simulink model "Furnace"  (R2020a)
settings: Solver=ode15s  StartTime=0  StopTime=27000  FixedStep=0.1  MaxStep=20  MinStep=1e-13  RelTol=1e-08  AbsTol=1e-09
undefined symbols (not defined in the file): agnostic_lqe_params, cont_reg, disturbance_type, F_aI_pid, F_aII_pid, input_type, k, lqe_params, LQR_params, LQRAgnostic_params, MPC_type, MPCDiscrete_function_parameters, MPCDiscreteAgnostic_function_parameters, MPCDiscreteDiffIntegralAgnostic_function_parameters, original_LQR_params, output_type, reg, single_butter_ss
libraries: simulink x35, cstblocks x10, mpclib x3
(part 5 of 8)

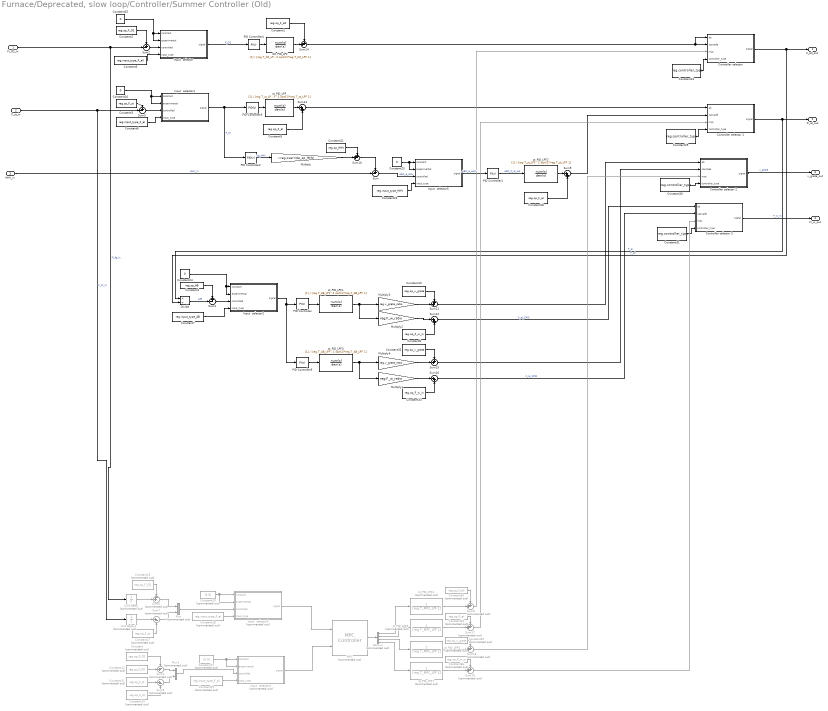
== system Furnace/Deprecated, slow loop/Controller/Summer Controller (Old)  ==
  Fi_O2_in : Inport
  F_st_in : Inport  Port=2
  HHV_in : Inport  Port=3
  Constant : Constant  Commented=on  Value=reg.op_F_O2
  Constant1 : Constant  Value=reg.op_F_aII
  Constant10 : Constant  Value=reg.op_v_grate
  Constant11 : Constant  Commented=on  Value=reg.sp_F_st
  Constant12 : Constant  Commented=on  Value=reg.sp_F_O2
  Constant{13,29..31} (4 alike) : Constant  Value=reg.controller_type
  Constant14 : Constant  Commented=on  Value=reg.op_F_st
  Constant15 : Constant  Commented=on  Value=reg.op_F_aI
  Constant16 : Constant  Commented=on  Value=reg.op_F_O2
  Constant17 : Constant  Commented=on  Value=reg.op_F_st
  Constant18 : Constant  Commented=on  Value=reg.input_type_F_aI
  Constant19 : Constant  Commented=on  Value=reg.input_type_F_aI
  Constant2 : Constant  Value=reg.sp_F_O2
  Constant20 : Constant  Commented=on  Value=[0 0]
  Constant21 : Constant  Value=reg.op_HHV
  Constant22 : Constant  Value=reg.input_type_HHV
  Constant{23..26} (4 alike) : Constant  Value=0
  Constant27 : Constant  Commented=on  Value=[0 0]
  Constant28 : Constant  Value=reg.op_F_aI
  Constant3 : Constant  Value=reg.sp_F_st
  Constant32 : Constant  Value=reg.op_v_grate
  Constant33 : Constant  Value=reg.op_F_w_in
  Constant34 : Constant  Commented=on  Value=reg.op_F_aII
  Constant35 : Constant  Commented=on  Value=reg.op_v_grate
  Constant36 : Constant  Commented=on  Value=reg.op_F_w_in
  Constant4 : Constant  Value=reg.sp_AB
  Constant5 : Constant  Value=reg.input_type_F_aII
  Constant6 : Constant  Value=reg.input_type_F_aI
  Constant7 : Constant  Value=reg.input_type_AB
  Constant8 : Constant  Value=reg.op_F_w_in
  Constant9 : Constant  Value=reg.op_F_aI
  "Controller selector " : MATLAB Function  TreatAsAtomicUnit=on
  Controller selector 1 : MATLAB Function  TreatAsAtomicUnit=on
  Controller selector 2 : MATLAB Function  TreatAsAtomicUnit=on
  Controller selector 3 : MATLAB Function  TreatAsAtomicUnit=on
  Demux : Demux  Commented=on
  Divide : Product  Inputs=*/  OutMin=[-100]  OutMax=[100]
  Input  selector : MATLAB Function  TreatAsAtomicUnit=on
  Input  selector1 : MATLAB Function  TreatAsAtomicUnit=on
  Input  selector2 : MATLAB Function  TreatAsAtomicUnit=on
  Input  selector3 : MATLAB Function  Commented=on  TreatAsAtomicUnit=on
  Input  selector4 : MATLAB Function  Commented=on  TreatAsAtomicUnit=on
  Input  selector5 : MATLAB Function  TreatAsAtomicUnit=on
  MPC : mpclib/MPC Controller  Commented=on  SCDEnableBlockLinearizationSpecification=on  mpcobj=lmpc  is_multiple=0  enable_value=0  return_u0=off  updateMPCinCallerWorkspace=on  md_inport=off  mv_inport=off  uref_inport=off  return_cost=off  return_mvseq=off  return_qpstatus=off  return_xseq=off  return_state=off  return_ovseq=off  state_inport=off  umin_inport=off  umax_inport=off  ymin_inport=off  ymax_inport=off  cc_inport=off  ywt_inport=off  uwt_inport=off  duwt_inport=off  rhoeps_inport=off  pm_inport=off  MaximumP=10  HorizonChoice=FixedHorizon  n_ts=20  n_p=50  n_mv=4  n_md=0  n_ud=0  n_mo=2  n_uo=0  BlockDataType=double  SampleTimeInherited=off  switch_inport=off
  Multiply : Gain  Gain=~reg.override_sp_HHV
  Multiply1 : Gain  Gain=reg.F_w_ratio
  Multiply2 : Gain  Gain=reg.F_w_ratio
  Multiply3 : Gain  Gain=reg.v_grate_ratio
  Multiply4 : Gain  Gain=reg.v_grate_ratio
  Mux : Mux  Commented=on  Inputs=2
  Mux1 : Mux  Commented=on  Inputs=2
  O2_PID_LPF : TransferFcn  Denominator=[reg.T_O2_LPF^2 sqrt(2)*reg.T_O2_LPF 1]
  PID Controller : simulink/Continuous/PID Controller  Controller=PI  Form=Parallel  TimeDomain=Discrete-time  UseExternalTs=off  SampleTime=1  IntegratorMethod=Forward Euler  FilterMethod=Forward Euler  ControllerParametersSource=internal  P=reg.Kp_AB  I=reg.Ki_AB  D=0  UseFilter=on  N=100  TunerSelectOption=Transfer Function Based (PID Tuner App)  InitialConditionSource=internal  InitialConditionForIntegrator=0  InitialConditionForFilter=0  DifferentiatorICPrevScaledInput=0  ExternalReset=none  TrackingMode=off  Kt=1  LimitOutput=off  UpperSaturationLimit=inf  LowerSaturationLimit=-inf  LinearizeAsGain=on  AntiWindupMode=none  Kb=1  POutMin=[]  POutMax=[]  IOutMin=[]  IOutMax=[]  DOutMin=[]  DOutMax=[]  NOutMin=[]  NOutMax=[]  SumOutMin=[]  SumOutMax=[]  SaturationOutMin=[]  SaturationOutMax=[]  PParamMin=[]  PParamMax=[]  IParamMin=[]  IParamMax=[]  DParamMin=[]  DParamMax=[]  NParamMin=[]  NParamMax=[]  KbParamMin=[]  KbParamMax=[]  KtParamMin=[]  KtParamMax=[]  KbOutMin=[]  KbOutMax=[]  KtOutMin=[]  KtOutMax=[]  IntegratorOutMin=[]  IntegratorOutMax=[]  FilterOutMin=[]  FilterOutMax=[]  SumI1OutMin=[]  SumI1OutMax=[]  SumI2OutMin=[]  SumI2OutMax=[]  SumI3OutMin=[]  SumI3OutMax=[]  SumI4OutMin=[]  SumI4OutMax=[]  SumDOutMin=[]  SumDOutMax=[]  DifferentiatorOutMin=[]  DifferentiatorOutMax=[]  FilterDiffOutCoefMin=[]  FilterDiffOutCoefMax=[]  ReciprocalOutMin=[]  ReciprocalOutMax=[]  SumDenOutMin=[]  SumDenOutMax=[]  SumNumOutMin=[]  SumNumOutMax=[]  DivideOutMin=[]  DivideOutMax=[]  UdiffTsProdOutMin=[]  UdiffTsProdOutMax=[]  NTsProdOutMin=[]  NTsProdOutMax=[]  UintegralTsProdOutMin=[]  UintegralTsProdOutMax=[]  UngainTsProdOutMin=[]  UngainTsProdOutMax=[]  IntegratorContinuousStateAttributes=''  IntegratorStateMustResolveToSignalObject=off  IntegratorRTWStateStorageClass=Auto  FilterContinuousStateAttributes=''  FilterStateMustResolveToSignalObject=off  FilterRTWStateStorageClass=Auto  ParallelPVariant=InternalParameters  IdealPVariant=Disabled  IVariant=InternalParameters  DVariant=Disabled  IntegratorVariant=Discrete  SatVariant=Disabled  AWVariant=Passthrough  PCopyVariant=Disabled  TRVariant=Disabled  FdbkBlocksVariant=Forward  IdealPFdbkVariant=Disabled  SatFdbkVariant=Disabled  DerivativeFilterVariant=Disabled  NVariant=Disabled  NCopyVariant=Disabled_SignalSpec  FilterICVariant=Disabled  IntegratorICVariant=InternalICs  ExternalResetVariant=Disabled  TRSumVariant=Passthrough  SumFdbkVariant=Disabled  SumVariant=Sum_PI  TsampFilterVariant=InternalTs  TsampNgainVariant=Passthrough  TsampIntegralVariant=Passthrough
  PID Controller1 : simulink/Continuous/PID Controller  Controller=PI  Form=Parallel  TimeDomain=Discrete-time  UseExternalTs=off  SampleTime=1  IntegratorMethod=Forward Euler  FilterMethod=Forward Euler  ControllerParametersSource=internal  P=reg.Kp_HHV  I=reg.Ki_HHV  D=0  UseFilter=on  N=100  TunerSelectOption=Transfer Function Based (PID Tuner App)  InitialConditionSource=internal  InitialConditionForIntegrator=0  InitialConditionForFilter=0  DifferentiatorICPrevScaledInput=0  ExternalReset=none  TrackingMode=off  Kt=1  LimitOutput=off  UpperSaturationLimit=inf  LowerSaturationLimit=-inf  LinearizeAsGain=on  AntiWindupMode=none  Kb=1  POutMin=[]  POutMax=[]  IOutMin=[]  IOutMax=[]  DOutMin=[]  DOutMax=[]  NOutMin=[]  NOutMax=[]  SumOutMin=[]  SumOutMax=[]  SaturationOutMin=[]  SaturationOutMax=[]  PParamMin=[]  PParamMax=[]  IParamMin=[]  IParamMax=[]  DParamMin=[]  DParamMax=[]  NParamMin=[]  NParamMax=[]  KbParamMin=[]  KbParamMax=[]  KtParamMin=[]  KtParamMax=[]  KbOutMin=[]  KbOutMax=[]  KtOutMin=[]  KtOutMax=[]  IntegratorOutMin=[]  IntegratorOutMax=[]  FilterOutMin=[]  FilterOutMax=[]  SumI1OutMin=[]  SumI1OutMax=[]  SumI2OutMin=[]  SumI2OutMax=[]  SumI3OutMin=[]  SumI3OutMax=[]  SumI4OutMin=[]  SumI4OutMax=[]  SumDOutMin=[]  SumDOutMax=[]  DifferentiatorOutMin=[]  DifferentiatorOutMax=[]  FilterDiffOutCoefMin=[]  FilterDiffOutCoefMax=[]  ReciprocalOutMin=[]  ReciprocalOutMax=[]  SumDenOutMin=[]  SumDenOutMax=[]  SumNumOutMin=[]  SumNumOutMax=[]  DivideOutMin=[]  DivideOutMax=[]  UdiffTsProdOutMin=[]  UdiffTsProdOutMax=[]  NTsProdOutMin=[]  NTsProdOutMax=[]  UintegralTsProdOutMin=[]  UintegralTsProdOutMax=[]  UngainTsProdOutMin=[]  UngainTsProdOutMax=[]  IntegratorContinuousStateAttributes=''  IntegratorStateMustResolveToSignalObject=off  IntegratorRTWStateStorageClass=Auto  FilterContinuousStateAttributes=''  FilterStateMustResolveToSignalObject=off  FilterRTWStateStorageClass=Auto  ParallelPVariant=InternalParameters  IdealPVariant=Disabled  IVariant=InternalParameters  DVariant=Disabled  IntegratorVariant=Discrete  SatVariant=Disabled  AWVariant=Passthrough  PCopyVariant=Disabled  TRVariant=Disabled  FdbkBlocksVariant=Forward  IdealPFdbkVariant=Disabled  SatFdbkVariant=Disabled  DerivativeFilterVariant=Disabled  NVariant=Disabled  NCopyVariant=Disabled_SignalSpec  FilterICVariant=Disabled  IntegratorICVariant=InternalICs  ExternalResetVariant=Disabled  TRSumVariant=Passthrough  SumFdbkVariant=Disabled  SumVariant=Sum_PI  TsampFilterVariant=InternalTs  TsampNgainVariant=Passthrough  TsampIntegralVariant=Passthrough
  PID Controller2 : simulink/Continuous/PID Controller  Controller=PID  Form=Parallel  TimeDomain=Discrete-time  UseExternalTs=off  SampleTime=1  IntegratorMethod=Forward Euler  FilterMethod=Forward Euler  ControllerParametersSource=internal  P=reg.Kp_st_HHV  I=reg.Ki_st_HHV  D=reg.Kd_st_HHV  UseFilter=on  N=100  TunerSelectOption=Transfer Function Based (PID Tuner App)  InitialConditionSource=internal  InitialConditionForIntegrator=0.001  InitialConditionForFilter=0  DifferentiatorICPrevScaledInput=0  ExternalReset=none  TrackingMode=off  Kt=1  LimitOutput=off  UpperSaturationLimit=inf  LowerSaturationLimit=1  LinearizeAsGain=on  AntiWindupMode=none  Kb=1  POutMin=[]  POutMax=[]  IOutMin=[]  IOutMax=[]  DOutMin=[]  DOutMax=[]  NOutMin=[]  NOutMax=[]  SumOutMin=[]  SumOutMax=[]  SaturationOutMin=[]  SaturationOutMax=[]  PParamMin=[]  PParamMax=[]  IParamMin=[]  IParamMax=[]  DParamMin=[]  DParamMax=[]  NParamMin=[]  NParamMax=[]  KbParamMin=[]  KbParamMax=[]  KtParamMin=[]  KtParamMax=[]  KbOutMin=[]  KbOutMax=[]  KtOutMin=[]  KtOutMax=[]  IntegratorOutMin=[]  IntegratorOutMax=[]  FilterOutMin=[]  FilterOutMax=[]  SumI1OutMin=[]  SumI1OutMax=[]  SumI2OutMin=[]  SumI2OutMax=[]  SumI3OutMin=[]  SumI3OutMax=[]  SumI4OutMin=[]  SumI4OutMax=[]  SumDOutMin=[]  SumDOutMax=[]  DifferentiatorOutMin=[]  DifferentiatorOutMax=[]  FilterDiffOutCoefMin=[]  FilterDiffOutCoefMax=[]  ReciprocalOutMin=[]  ReciprocalOutMax=[]  SumDenOutMin=[]  SumDenOutMax=[]  SumNumOutMin=[]  SumNumOutMax=[]  DivideOutMin=[]  DivideOutMax=[]  UdiffTsProdOutMin=[]  UdiffTsProdOutMax=[]  NTsProdOutMin=[]  NTsProdOutMax=[]  UintegralTsProdOutMin=[]  UintegralTsProdOutMax=[]  UngainTsProdOutMin=[]  UngainTsProdOutMax=[]  IntegratorContinuousStateAttributes='F_st'  IntegratorStateMustResolveToSignalObject=off  IntegratorRTWStateStorageClass=Auto  FilterContinuousStateAttributes=''  FilterStateMustResolveToSignalObject=off  FilterRTWStateStorageClass=Auto  ParallelPVariant=InternalParameters  IdealPVariant=Disabled  IVariant=InternalParameters  DVariant=InternalParameters  IntegratorVariant=Discrete  SatVariant=Disabled  AWVariant=Passthrough  PCopyVariant=Disabled  TRVariant=Disabled  FdbkBlocksVariant=Forward  IdealPFdbkVariant=Disabled  SatFdbkVariant=Disabled  DerivativeFilterVariant=ForwardEulerFilter  NVariant=InternalParameters  NCopyVariant=Disabled  FilterICVariant=InternalICsFilter  IntegratorICVariant=InternalICs  ExternalResetVariant=Disabled  TRSumVariant=Passthrough  SumFdbkVariant=Disabled  SumVariant=Sum_PID  TsampFilterVariant=InternalTs  TsampNgainVariant=Passthrough  TsampIntegralVariant=Passthrough
  PID Controller3 : simulink/Continuous/PID Controller  Controller=PID  Form=Parallel  TimeDomain=Discrete-time  UseExternalTs=off  SampleTime=1  IntegratorMethod=Forward Euler  FilterMethod=Forward Euler  ControllerParametersSource=internal  P=reg.Kp_st  I=reg.Ki_st  D=reg.Kd_st  UseFilter=on  N=100  TunerSelectOption=Transfer Function Based (PID Tuner App)  InitialConditionSource=internal  InitialConditionForIntegrator=0  InitialConditionForFilter=0  DifferentiatorICPrevScaledInput=0  ExternalReset=none  TrackingMode=off  Kt=1  LimitOutput=off  UpperSaturationLimit=inf  LowerSaturationLimit=1  LinearizeAsGain=on  AntiWindupMode=none  Kb=1  POutMin=[]  POutMax=[]  IOutMin=[]  IOutMax=[]  DOutMin=[]  DOutMax=[]  NOutMin=[]  NOutMax=[]  SumOutMin=[]  SumOutMax=[]  SaturationOutMin=[]  SaturationOutMax=[]  PParamMin=[]  PParamMax=[]  IParamMin=[]  IParamMax=[]  DParamMin=[]  DParamMax=[]  NParamMin=[]  NParamMax=[]  KbParamMin=[]  KbParamMax=[]  KtParamMin=[]  KtParamMax=[]  KbOutMin=[]  KbOutMax=[]  KtOutMin=[]  KtOutMax=[]  IntegratorOutMin=[]  IntegratorOutMax=[]  FilterOutMin=[]  FilterOutMax=[]  SumI1OutMin=[]  SumI1OutMax=[]  SumI2OutMin=[]  SumI2OutMax=[]  SumI3OutMin=[]  SumI3OutMax=[]  SumI4OutMin=[]  SumI4OutMax=[]  SumDOutMin=[]  SumDOutMax=[]  DifferentiatorOutMin=[]  DifferentiatorOutMax=[]  FilterDiffOutCoefMin=[]  FilterDiffOutCoefMax=[]  ReciprocalOutMin=[]  ReciprocalOutMax=[]  SumDenOutMin=[]  SumDenOutMax=[]  SumNumOutMin=[]  SumNumOutMax=[]  DivideOutMin=[]  DivideOutMax=[]  UdiffTsProdOutMin=[]  UdiffTsProdOutMax=[]  NTsProdOutMin=[]  NTsProdOutMax=[]  UintegralTsProdOutMin=[]  UintegralTsProdOutMax=[]  UngainTsProdOutMin=[]  UngainTsProdOutMax=[]  IntegratorContinuousStateAttributes='F_st'  IntegratorStateMustResolveToSignalObject=off  IntegratorRTWStateStorageClass=Auto  FilterContinuousStateAttributes=''  FilterStateMustResolveToSignalObject=off  FilterRTWStateStorageClass=Auto  ParallelPVariant=InternalParameters  IdealPVariant=Disabled  IVariant=InternalParameters  DVariant=InternalParameters  IntegratorVariant=Discrete  SatVariant=Disabled  AWVariant=Passthrough  PCopyVariant=Disabled  TRVariant=Disabled  FdbkBlocksVariant=Forward  IdealPFdbkVariant=Disabled  SatFdbkVariant=Disabled  DerivativeFilterVariant=ForwardEulerFilter  NVariant=InternalParameters  NCopyVariant=Disabled  FilterICVariant=InternalICsFilter  IntegratorICVariant=InternalICs  ExternalResetVariant=Disabled  TRSumVariant=Passthrough  SumFdbkVariant=Disabled  SumVariant=Sum_PID  TsampFilterVariant=InternalTs  TsampNgainVariant=Passthrough  TsampIntegralVariant=Passthrough
  PID Controller4 : simulink/Continuous/PID Controller  Controller=PI  Form=Parallel  TimeDomain=Discrete-time  UseExternalTs=off  SampleTime=1  IntegratorMethod=Forward Euler  FilterMethod=Forward Euler  ControllerParametersSource=internal  P=reg.Kp_O2  I=reg.Ki_O2  D=0  UseFilter=on  N=100  TunerSelectOption=Transfer Function Based (PID Tuner App)  InitialConditionSource=internal  InitialConditionForIntegrator=0.001  InitialConditionForFilter=0  DifferentiatorICPrevScaledInput=0  ExternalReset=none  TrackingMode=off  Kt=1  LimitOutput=off  UpperSaturationLimit=inf  LowerSaturationLimit=1  LinearizeAsGain=on  AntiWindupMode=none  Kb=1  POutMin=[]  POutMax=[]  IOutMin=[]  IOutMax=[]  DOutMin=[]  DOutMax=[]  NOutMin=[]  NOutMax=[]  SumOutMin=[]  SumOutMax=[]  SaturationOutMin=[]  SaturationOutMax=[]  PParamMin=[]  PParamMax=[]  IParamMin=[]  IParamMax=[]  DParamMin=[]  DParamMax=[]  NParamMin=[]  NParamMax=[]  KbParamMin=[]  KbParamMax=[]  KtParamMin=[]  KtParamMax=[]  KbOutMin=[]  KbOutMax=[]  KtOutMin=[]  KtOutMax=[]  IntegratorOutMin=[]  IntegratorOutMax=[]  FilterOutMin=[]  FilterOutMax=[]  SumI1OutMin=[]  SumI1OutMax=[]  SumI2OutMin=[]  SumI2OutMax=[]  SumI3OutMin=[]  SumI3OutMax=[]  SumI4OutMin=[]  SumI4OutMax=[]  SumDOutMin=[]  SumDOutMax=[]  DifferentiatorOutMin=[]  DifferentiatorOutMax=[]  FilterDiffOutCoefMin=[]  FilterDiffOutCoefMax=[]  ReciprocalOutMin=[]  ReciprocalOutMax=[]  SumDenOutMin=[]  SumDenOutMax=[]  SumNumOutMin=[]  SumNumOutMax=[]  DivideOutMin=[]  DivideOutMax=[]  UdiffTsProdOutMin=[]  UdiffTsProdOutMax=[]  NTsProdOutMin=[]  NTsProdOutMax=[]  UintegralTsProdOutMin=[]  UintegralTsProdOutMax=[]  UngainTsProdOutMin=[]  UngainTsProdOutMax=[]  IntegratorContinuousStateAttributes='F_st'  IntegratorStateMustResolveToSignalObject=off  IntegratorRTWStateStorageClass=Auto  FilterContinuousStateAttributes=''  FilterStateMustResolveToSignalObject=off  FilterRTWStateStorageClass=Auto  ParallelPVariant=InternalParameters  IdealPVariant=Disabled  IVariant=InternalParameters  DVariant=Disabled  IntegratorVariant=Discrete  SatVariant=Disabled  AWVariant=Passthrough  PCopyVariant=Disabled  TRVariant=Disabled  FdbkBlocksVariant=Forward  IdealPFdbkVariant=Disabled  SatFdbkVariant=Disabled  DerivativeFilterVariant=Disabled  NVariant=Disabled  NCopyVariant=Disabled_SignalSpec  FilterICVariant=Disabled  IntegratorICVariant=InternalICs  ExternalResetVariant=Disabled  TRSumVariant=Passthrough  SumFdbkVariant=Disabled  SumVariant=Sum_PI  TsampFilterVariant=InternalTs  TsampNgainVariant=Passthrough  TsampIntegralVariant=Passthrough
  PID Controller5 : simulink/Continuous/PID Controller  Controller=PI  Form=Parallel  TimeDomain=Discrete-time  UseExternalTs=off  SampleTime=1  IntegratorMethod=Forward Euler  FilterMethod=Forward Euler  ControllerParametersSource=internal  P=reg.Kp_AB_HHV  I=reg.Ki_AB_HHV  D=0  UseFilter=on  N=100  TunerSelectOption=Transfer Function Based (PID Tuner App)  InitialConditionSource=internal  InitialConditionForIntegrator=0  InitialConditionForFilter=0  DifferentiatorICPrevScaledInput=0  ExternalReset=none  TrackingMode=off  Kt=1  LimitOutput=off  UpperSaturationLimit=inf  LowerSaturationLimit=-inf  LinearizeAsGain=on  AntiWindupMode=none  Kb=1  POutMin=[]  POutMax=[]  IOutMin=[]  IOutMax=[]  DOutMin=[]  DOutMax=[]  NOutMin=[]  NOutMax=[]  SumOutMin=[]  SumOutMax=[]  SaturationOutMin=[]  SaturationOutMax=[]  PParamMin=[]  PParamMax=[]  IParamMin=[]  IParamMax=[]  DParamMin=[]  DParamMax=[]  NParamMin=[]  NParamMax=[]  KbParamMin=[]  KbParamMax=[]  KtParamMin=[]  KtParamMax=[]  KbOutMin=[]  KbOutMax=[]  KtOutMin=[]  KtOutMax=[]  IntegratorOutMin=[]  IntegratorOutMax=[]  FilterOutMin=[]  FilterOutMax=[]  SumI1OutMin=[]  SumI1OutMax=[]  SumI2OutMin=[]  SumI2OutMax=[]  SumI3OutMin=[]  SumI3OutMax=[]  SumI4OutMin=[]  SumI4OutMax=[]  SumDOutMin=[]  SumDOutMax=[]  DifferentiatorOutMin=[]  DifferentiatorOutMax=[]  FilterDiffOutCoefMin=[]  FilterDiffOutCoefMax=[]  ReciprocalOutMin=[]  ReciprocalOutMax=[]  SumDenOutMin=[]  SumDenOutMax=[]  SumNumOutMin=[]  SumNumOutMax=[]  DivideOutMin=[]  DivideOutMax=[]  UdiffTsProdOutMin=[]  UdiffTsProdOutMax=[]  NTsProdOutMin=[]  NTsProdOutMax=[]  UintegralTsProdOutMin=[]  UintegralTsProdOutMax=[]  UngainTsProdOutMin=[]  UngainTsProdOutMax=[]  IntegratorContinuousStateAttributes=''  IntegratorStateMustResolveToSignalObject=off  IntegratorRTWStateStorageClass=Auto  FilterContinuousStateAttributes=''  FilterStateMustResolveToSignalObject=off  FilterRTWStateStorageClass=Auto  ParallelPVariant=InternalParameters  IdealPVariant=Disabled  IVariant=InternalParameters  DVariant=Disabled  IntegratorVariant=Discrete  SatVariant=Disabled  AWVariant=Passthrough  PCopyVariant=Disabled  TRVariant=Disabled  FdbkBlocksVariant=Forward  IdealPFdbkVariant=Disabled  SatFdbkVariant=Disabled  DerivativeFilterVariant=Disabled  NVariant=Disabled  NCopyVariant=Disabled_SignalSpec  FilterICVariant=Disabled  IntegratorICVariant=InternalICs  ExternalResetVariant=Disabled  TRSumVariant=Passthrough  SumFdbkVariant=Disabled  SumVariant=Sum_PI  TsampFilterVariant=InternalTs  TsampNgainVariant=Passthrough  TsampIntegralVariant=Passthrough
  Sum{,2..4} (4 alike) : Sum  Inputs=+-|
  Sum1 : Sum  Commented=on  Inputs=-+|
  Sum{10..11,14..15} (4 alike) : Sum  Inputs=++|
  Sum{9,12..13,16} (4 alike) : Sum  Inputs=|++
  Sum{8,17..19} (4 alike) : Sum  Commented=on  Inputs=++|
  Sum5 : Sum  Commented=on  Inputs=|+-
  Sum6 : Sum  Commented=on  Inputs=-+|
  Sum7 : Sum  Commented=on  Inputs=|+-
  Unit Delay : UnitDelay  Commented=on  HasFrameUpgradeWarning=on
  Unit Delay1 : UnitDelay  Commented=on  HasFrameUpgradeWarning=on
  st_PID_LPF : TransferFcn  Denominator=[reg.T_st_LPF^2 sqrt(2)*reg.T_st_LPF 1]
  st_PID_LPF1 : TransferFcn  Denominator=[reg.T_AB_LPF^2 sqrt(2)*reg.T_AB_LPF 1]
  st_PID_LPF2 : TransferFcn  Denominator=[reg.T_st_LPF^2 sqrt(2)*reg.T_st_LPF 1]
  st_PID_LPF3 : TransferFcn  Denominator=[reg.T_AB_LPF^2 sqrt(2)*reg.T_AB_LPF 1]
  st_PID_LPF{4..7} (4 alike) : TransferFcn  Commented=on  Denominator=[reg.T_MPC_LPF 1]
  F_aII_out : Outport  VectorParamsAs1DForOutWhenUnconnected=off
  Fi_aI_out : Outport  Port=2  VectorParamsAs1DForOutWhenUnconnected=off
  v_grate_out : Outport  Port=3  VectorParamsAs1DForOutWhenUnconnected=off
  Fi_w_out : Outport  Port=4  VectorParamsAs1DForOutWhenUnconnected=off
  wires:
  Input  selector/1(signal) -> PID Controller4/1  "F_O2"
  Constant7/1 -> Input  selector2/4(input_type)
  Constant5/1 -> Input  selector/4(input_type)
  Constant4/1 -> Sum4/1
  Fi_O2_in/1 -> Unit Delay/1, Sum2/2  "Fi_fg_in"
  Constant2/1 -> Sum2/1
  F_st_in/1 -> Sum3/2, Unit Delay1/1  "F_st_in"
  Constant3/1 -> Sum3/1
  PID Controller4/1 -> O2_PID_LPF/1
  Sum14/1 -> "Controller selector "/1(ab), "Controller selector "/2(cascade)
  PID Controller3/1 -> st_PID_LPF/1
  Sum13/1 -> Controller selector 1/1(ab)
  Constant8/1 -> Sum12/2
  PID Controller/1 -> st_PID_LPF1/1
  Sum11/1 -> Controller selector 2/1(ab)
  Multiply2/1 -> Sum12/1
  Constant10/1 -> Sum11/1
  st_PID_LPF/1 -> Sum13/1
  st_PID_LPF1/1 -> Multiply2/1, Multiply3/1
  Demux/1 -> st_PID_LPF4/1
  Demux/2 -> st_PID_LPF5/1
  Demux/3 -> st_PID_LPF6/1
  Demux/4 -> st_PID_LPF7/1
  "Controller selector "/1(signal) -> Divide/2, F_aII_out/1  "F_aII"
  Controller selector 1/1(signal) -> Divide/1, Fi_aI_out/1  "F_aI"
  Controller selector 2/1(signal) -> v_grate_out/1  "v_grate"
  Controller selector 3/1(signal) -> Fi_w_out/1  "F_w_in"
  Constant12/1 -> Sum1/2
  Constant/1 -> Sum1/1
  Constant11/1 -> Sum5/1
  Constant14/1 -> Sum5/2
  Sum5/1 -> Mux1/2
  MPC/1 -> Demux/1
  Sum7/1 -> Mux/2
  Constant16/1 -> Sum6/1
  Constant17/1 -> Sum7/2
  Input  selector3/1(signal) -> MPC/1
  Mux/1 -> Input  selector3/3(controlled)
  Constant18/1 -> Input  selector3/4(input_type)
  Constant19/1 -> Input  selector4/4(input_type)
  Mux1/1 -> Input  selector4/3(controlled)
  Input  selector4/1(signal) -> MPC/2
  Constant20/1 -> Input  selector3/2(experimental), Input  selector3/1(constant)
  HHV_in/1 -> Sum/2  "HHV_in"
  Input  selector5/1(signal) -> PID Controller1/1  "ABC_e_HHV"
  Constant22/1 -> Input  selector5/4(input_type)
  Sum/1 -> Input  selector5/3(controlled)  "ABC_e_HHV"
  Constant23/1 -> Input  selector5/2(experimental), Input  selector5/1(constant)
  Divide/1 -> Sum4/2  "A/B"
  Sum4/1 -> Input  selector2/3(controlled)
  Input  selector2/1(signal) -> PID Controller5/1, PID Controller/1
  Constant24/1 -> Input  selector2/2(experimental), Input  selector2/1(constant)
  Sum2/1 -> Input  selector/3(controlled)
  Constant25/1 -> Input  selector/2(experimental), Input  selector/1(constant)
  Sum3/1 -> Input  selector1/3(controlled)
  Constant6/1 -> Input  selector1/4(input_type)
  Constant26/1 -> Input  selector1/2(experimental), Input  selector1/1(constant)
  Input  selector1/1(signal) -> PID Controller3/1, PID Controller2/1  "F_st"
  Constant27/1 -> Input  selector4/2(experimental), Input  selector4/1(constant)
  Sum12/1 -> Controller selector 3/1(ab)  "F_aI_CPID"
  PID Controller1/1 -> st_PID_LPF2/1  "ABC_F_aI_out"
  Sum9/1 -> Controller selector 1/2(cascade)
  PID Controller2/1 -> Multiply/1  "sp_HHV"
  Multiply/1 -> Sum10/2
  Constant21/1 -> Sum10/1
  Sum10/1 -> Sum/1
  st_PID_LPF2/1 -> Sum9/1
  Sum1/1 -> Mux1/1
  Sum6/1 -> Mux/1
  Constant28/1 -> Sum9/2
  Constant9/1 -> Sum13/2
  O2_PID_LPF/1 -> Sum14/2
  Constant1/1 -> Sum14/1
  Constant13/1 -> "Controller selector "/4(controller_type)
  Constant29/1 -> Controller selector 1/4(controller_type)
  Constant30/1 -> Controller selector 2/4(controller_type)
  Constant31/1 -> Controller selector 3/4(controller_type)
  st_PID_LPF3/1 -> Multiply1/1, Multiply4/1
  PID Controller5/1 -> st_PID_LPF3/1
  Constant33/1 -> Sum16/2
  Constant32/1 -> Sum15/1
  Multiply1/1 -> Sum16/1
  Sum15/1 -> Controller selector 2/2(cascade)
  Sum16/1 -> Controller selector 3/2(cascade)  "F_aI_CPID"
  Unit Delay/1 -> Sum6/2
  Unit Delay1/1 -> Sum7/1
  st_PID_LPF4/1 -> Sum8/2
  st_PID_LPF5/1 -> Sum17/2
  st_PID_LPF6/1 -> Sum18/2
  st_PID_LPF7/1 -> Sum19/2
  Constant34/1 -> Sum8/1
  Constant15/1 -> Sum17/1
  Constant35/1 -> Sum18/1
  Constant36/1 -> Sum19/1
  Sum17/1 -> Controller selector 1/3(mpc)
  Sum8/1 -> "Controller selector "/3(mpc)
  Sum18/1 -> Controller selector 2/3(mpc)
  Sum19/1 -> Controller selector 3/3(mpc)
  Multiply3/1 -> Sum11/2
  Multiply4/1 -> Sum15/2

== system Furnace/Deprecated, slow loop/Furnace/Ashes ==
  In1 : Inport
  In2 : Inport  Port=2
  In Bus Element : Inport  Port=3  PortName=InBus  Element=M_w_grate
  In Bus Element1 : Inport  Port=3  PortName=InBus  Element=M_char
  In Bus Element2 : Inport  Port=3  PortName=InBus  Element=F_w_ash
  In Bus Element3 : Inport  Port=3  PortName=InBus  Element=F_char_ash
  Flow of char ash : Display
  Flow of waste ash : Display
  Mass of char in grate : Display
  Scope1 : Scope
  Sum of Elements : Sum  Inputs=+  CollapseMode=Specified dimension
  Temperatures in grate : Display
  Waste in grate (mass) : Display
  wires:
  In Bus Element2/1 -> Flow of waste ash/1
  In Bus Element/1 -> Waste in grate (mass)/1
  In Bus Element1/1 -> Mass of char in grate/1
  In Bus Element3/1 -> Flow of char ash/1
  In1/1 -> Sum of Elements/1
  In2/1 -> Temperatures in grate/1
  Sum of Elements/1 -> Scope1/1

== system Furnace/Deprecated, slow loop/Furnace/Auxiliary "burners" ==
  In1 : Inport
  Constant : Constant  Value=0
  Constant1 : Constant  Value=850+k.T_amb
  Minus : Sum  Inputs=+-
  "Q " : Constant  Value=3.5e6
  Switch : Switch  Criteria=u2 > Threshold
  Out1 : Outport  VectorParamsAs1DForOutWhenUnconnected=off
  wires:
  Switch/1 -> Out1/1
  Constant/1 -> Switch/3
  "Q "/1 -> Switch/1
  Minus/1 -> Switch/2
  Constant1/1 -> Minus/1
  In1/1 -> Minus/2

== system Furnace/Deprecated, slow loop/Furnace/Boiler ==
  T_fromHE : Inport
  T_fg : Inport  Port=2
  F_fg : Inport  Port=3
  F_flyash : Inport  Port=4
  F_ECO : Inport  Port=5
  Constant : Constant  Value=0
  Constant1 : Constant  Value=k.p_drum
  Constant2 : Constant  Value=k.p_drum
  Drum : Subsystem
      mask Display: image('Drum.jpg');
  Economizer : Subsystem
  Evaporator : Subsystem
  Gain : Gain  Gain=1e-5
  Goto : Goto  Commented=on  GotoTag=T_drum  TagVisibility=global
  MATLAB Function : MATLAB Function  TreatAsAtomicUnit=on
  PID Controller : simulink/Continuous/PID Controller  Controller=PID  Form=Parallel  TimeDomain=Continuous-time  UseExternalTs=off  SampleTime=-1  IntegratorMethod=Forward Euler  FilterMethod=Forward Euler  ControllerParametersSource=internal  P=10  I=0  D=0  UseFilter=on  N=100  TunerSelectOption=Transfer Function Based (PID Tuner App)  InitialConditionSource=internal  InitialConditionForIntegrator=0  InitialConditionForFilter=0  DifferentiatorICPrevScaledInput=0  ExternalReset=none  TrackingMode=off  Kt=1  LimitOutput=on  UpperSaturationLimit=50  LowerSaturationLimit=0  LinearizeAsGain=on  AntiWindupMode=none  Kb=1  POutMin=[]  POutMax=[]  IOutMin=[]  IOutMax=[]  DOutMin=[]  DOutMax=[]  NOutMin=[]  NOutMax=[]  SumOutMin=[]  SumOutMax=[]  SaturationOutMin=[]  SaturationOutMax=[]  PParamMin=[]  PParamMax=[]  IParamMin=[]  IParamMax=[]  DParamMin=[]  DParamMax=[]  NParamMin=[]  NParamMax=[]  KbParamMin=[]  KbParamMax=[]  KtParamMin=[]  KtParamMax=[]  KbOutMin=[]  KbOutMax=[]  KtOutMin=[]  KtOutMax=[]  IntegratorOutMin=[]  IntegratorOutMax=[]  FilterOutMin=[]  FilterOutMax=[]  SumI1OutMin=[]  SumI1OutMax=[]  SumI2OutMin=[]  SumI2OutMax=[]  SumI3OutMin=[]  SumI3OutMax=[]  SumI4OutMin=[]  SumI4OutMax=[]  SumDOutMin=[]  SumDOutMax=[]  DifferentiatorOutMin=[]  DifferentiatorOutMax=[]  FilterDiffOutCoefMin=[]  FilterDiffOutCoefMax=[]  ReciprocalOutMin=[]  ReciprocalOutMax=[]  SumDenOutMin=[]  SumDenOutMax=[]  SumNumOutMin=[]  SumNumOutMax=[]  DivideOutMin=[]  DivideOutMax=[]  UdiffTsProdOutMin=[]  UdiffTsProdOutMax=[]  NTsProdOutMin=[]  NTsProdOutMax=[]  UintegralTsProdOutMin=[]  UintegralTsProdOutMax=[]  UngainTsProdOutMin=[]  UngainTsProdOutMax=[]  IntegratorContinuousStateAttributes=''  IntegratorStateMustResolveToSignalObject=off  IntegratorRTWStateStorageClass=Auto  FilterContinuousStateAttributes=''  FilterStateMustResolveToSignalObject=off  FilterRTWStateStorageClass=Auto  ParallelPVariant=InternalParameters  IdealPVariant=Disabled  IVariant=InternalParameters  DVariant=InternalParameters  IntegratorVariant=Continuous  SatVariant=Enabled  AWVariant=Passthrough  PCopyVariant=Disabled  TRVariant=Disabled  FdbkBlocksVariant=Forward  IdealPFdbkVariant=Disabled  SatFdbkVariant=Disabled  DerivativeFilterVariant=ContFilter  NVariant=InternalParameters  NCopyVariant=Disabled  FilterICVariant=InternalICsFilter  IntegratorICVariant=InternalICs  ExternalResetVariant=Disabled  TRSumVariant=Passthrough  SumFdbkVariant=Disabled  SumVariant=Sum_PID  TsampFilterVariant=InternalTs  TsampNgainVariant=Passthrough  TsampIntegralVariant=Passthrough
  PID null saturator : Switch
  Scope : Scope
  Scope1 : Scope
  Scope2 : Scope
  Sum1 : Sum  Inputs=+-|
  Super heater : Subsystem
  x_vap : Scope
  T_SH : Outport  VectorParamsAs1DForOutWhenUnconnected=off
  F_SH : Outport  Port=2  PortDimensions=1  VectorParamsAs1DForOutWhenUnconnected=off
  p_drum : Outport  Port=3  VectorParamsAs1DForOutWhenUnconnected=off
  T_fg_out : Outport  Port=4  VectorParamsAs1DForOutWhenUnconnected=off
  Fi_fg_out : Outport  Port=5  VectorParamsAs1DForOutWhenUnconnected=off
  F_flyash_out : Outport  Port=6  VectorParamsAs1DForOutWhenUnconnected=off
  wires:
  Evaporator/3(Fi_fg_out) -> Super heater/4(Fi_fg)
  Super heater/4(Fi_fg_out) -> Economizer/3(Fi_fg)
  Super heater/3(T_fg_out) -> Economizer/2(T_fg)
  Evaporator/2(T_fg_out) -> Super heater/3(T_fg)
  Economizer/3(Fi_fg_out) -> Fi_fg_out/1
  F_fg/1 -> Evaporator/3(Fi_fg)
  T_fg/1 -> Evaporator/2(T_fg)
  Super heater/2(T_steam) -> T_SH/1
  Economizer/2(T_fg_out) -> T_fg_out/1
  Drum/3(p_drum) -> MATLAB Function/1(p_drum), Sum1/1, p_drum/1
  T_fromHE/1 -> Economizer/1(T_fromHE)
  Super heater/5(F_SH) -> F_SH/1
  Drum/2(x_vap) -> x_vap/1
  PID Controller/1 -> Drum/3(F_vap), Scope/1, Super heater/1(F_steam)
  Constant1/1 -> Sum1/2
  Constant/1 -> PID null saturator/3
  Sum1/1 -> Gain/1
  [Q_cleaning] -> Drum/5(Q_cleaning)
  F_flyash/1 -> F_flyash_out/1
  Super heater/1(Q_SH) -> Scope1/1
  Economizer/1(Q_ECO) -> Scope2/1
  Economizer/4(F_ECO) -> Drum/1(F_ECO)
  Evaporator/1(Q_EVA) -> Drum/2(Q_EVA)
  Economizer/5(T_ECO2) -> Drum/4(T_ECO)
  F_ECO/1 -> Economizer/4(F_w)
  PID null saturator/1 -> PID Controller/1
  Gain/1 -> PID null saturator/1
  Drum/1(T_drum) -> Goto/1, Super heater/2(T_drum), Evaporator/1(T_drum)
  MATLAB Function/1(switch_on) -> PID null saturator/2
  Constant2/1 -> MATLAB Function/2(k_p_drum)

== system Furnace/Deprecated, slow loop/Furnace/Calorific Value ==
  T_fg : Inport
  Fi_fg : Inport  Port=2
  From : From  Commented=on  GotoTag=F_aII
  From1 : From  Commented=on  GotoTag=T_aI  TagVisibility=global
  From2 : From  Commented=on  GotoTag=F_aI  TagVisibility=global
  From3 : From  Commented=on  GotoTag=T_aII
  MATLAB Function : MATLAB Function  TreatAsAtomicUnit=on
  T_amb : Constant  Value=k.T_amb
  cp_fg : Constant  Value=k.cp_fg
  HHV : Outport  VectorParamsAs1DForOutWhenUnconnected=off
  wires:
  cp_fg/1 -> MATLAB Function/3(cp_fg)
  Fi_fg/1 -> MATLAB Function/1(Fi_fg)
  T_amb/1 -> MATLAB Function/4(T_amb)
  MATLAB Function/1(HHV) -> HHV/1
  T_fg/1 -> MATLAB Function/2(T_fg)
  From2/1 -> MATLAB Function/5(F_aI)
  From1/1 -> MATLAB Function/6(T_aI)
  From/1 -> MATLAB Function/7(F_aII)
  From3/1 -> MATLAB Function/8(T_aII)

== system Furnace/Deprecated, slow loop/Furnace/Cold water from district heating ==
  Constant : Constant  Value=reg.const_F_from_DH
  Constant2 : Constant  Value=reg.const_T_from_DH
  From Workspace1 : FromWorkspace  VariableName=F_from_DH
  From Workspace2 : FromWorkspace  VariableName=T_from_DH
  Selector : Selector  InputPortWidth=2  IndexOptions=Index vector (dialog)  Indices=reg.input_type_F_from_DH  OutputSizes=1
  Selector1 : Selector  InputPortWidth=2  IndexOptions=Index vector (dialog)  Indices=reg.input_type_T_from_DH  OutputSizes=1
  Vector Concatenate : Concatenate
  Vector Concatenate1 : Concatenate
  Out1 : Outport  VectorParamsAs1DForOutWhenUnconnected=off
  Out2 : Outport  Port=2  VectorParamsAs1DForOutWhenUnconnected=off
  wires:
  From Workspace1/1 -> Vector Concatenate/2
  Constant/1 -> Vector Concatenate/1
  Constant2/1 -> Vector Concatenate1/1
  From Workspace2/1 -> Vector Concatenate1/2
  Vector Concatenate/1 -> Selector/1
  Selector/1 -> Out1/1  "F_from_DH"
  Vector Concatenate1/1 -> Selector1/1
  Selector1/1 -> Out2/1  "T_from_DH"

== system Furnace/Deprecated, slow loop/Furnace/Condenser ==
  F_district : Inport
  F_turb : Inport  Port=2
  T_return : Inport  Port=3
  Constant : Constant  Value=k.cp_water
  Constant1 : Constant  Value=k.epsilon_HE
  Constant2 : Constant  Value=k.eff_HE
  District heating heat exchanger : MATLAB Function  TreatAsAtomicUnit=on
  Scope : Scope
  Transport Delay1 : TransportDelay  DelayTime=2
  Transport Delay2 : TransportDelay  DelayTime=2  InitialOutput=k.T_amb  BufferSize=2048
  Transport Delay3 : TransportDelay  DelayTime=2  InitialOutput=k.T_amb
  Transport Delay4 : TransportDelay  DelayTime=2  InitialOutput=k.T_amb
  p_HP : Constant  Value=k.p_HP
  T_district : Outport  VectorParamsAs1DForOutWhenUnconnected=off
  T_w_out : Outport  Port=2  VectorParamsAs1DForOutWhenUnconnected=off
  F_cond : Outport  Port=3  VectorParamsAs1DForOutWhenUnconnected=off
  wires:
  F_district/1 -> District heating heat exchanger/1(F_DH)
  p_HP/1 -> District heating heat exchanger/2(p_HP)
  T_return/1 -> District heating heat exchanger/4(T_return)
  Constant/1 -> District heating heat exchanger/5(cp_water)
  Constant1/1 -> District heating heat exchanger/6(epsilon_HE)
  District heating heat exchanger/1(Q_HE) -> Transport Delay1/1
  District heating heat exchanger/3(T_district) -> Transport Delay3/1
  District heating heat exchanger/2(Tw_ECO) -> Transport Delay2/1
  F_turb/1 -> Transport Delay4/1, District heating heat exchanger/3(F_turb)
  Transport Delay1/1 -> Scope/1
  Transport Delay2/1 -> T_w_out/1
  Transport Delay3/1 -> T_district/1
  Constant2/1 -> District heating heat exchanger/7(eff_HE)
  Transport Delay4/1 -> F_cond/1

== system Furnace/Deprecated, slow loop/Furnace/Flue-gas fan ==
  T_fg : Inport
  Fi_fg : Inport  Port=2
  Fan : MATLAB Function  TreatAsAtomicUnit=on
  Sum of Elements : Sum  Inputs=+
  Out1 : Outport  VectorParamsAs1DForOutWhenUnconnected=off
  Out2 : Outport  Port=2  VectorParamsAs1DForOutWhenUnconnected=off
  tag scope: W_fan=global
  wires:
  T_fg/1 -> Fan/1(T_fg)
  Sum of Elements/1 -> Fan/2(F_fg)
  Fi_fg/1 -> Out2/1, Sum of Elements/1
  Fan/1(T_out) -> Out1/1
  Fan/2(W_el) -> [W_fan]

== system Furnace/Deprecated, slow loop/Furnace/Flue-gas stack ==
  T_fg : Inport
  Fi_fg : Inport  Port=2
  F_fg : Scope
  T_fg_fromECO : Scope
  wires:
  T_fg/1 -> T_fg_fromECO/1
  Fi_fg/1 -> F_fg/1

== system Furnace/Deprecated, slow loop/Furnace/Free board ==
  Fi_in : Inport
  T_in : Inport  Port=2
  Q_rad : Inport  Port=3
  F_flyash_cell : Inport  Port=4
  F_aII_in : Inport  Port=5
  T_aII_in : Inport  Port=6
  DIFF_Free Board : MATLAB Function  TreatAsAtomicUnit=on
  M_fg_part : Integrator  InitialCondition=[k.M_fg_IC.*k.w_a(1:k.nc_gas-1)]
  M_steel : Constant  Value=k.M_steel_FB
  Mw_gas : Constant  Value=k.Mw_gas
  Scope : Scope
  Sum of Elements : Sum  Inputs=+
  T_amb : Constant  Value=k.T_amb
  T_fg : Integrator  InitialCondition=k.T_0
  To Workspace : ToWorkspace  Commented=on  VariableName=Y_H2O  SaveFormat=Structure With Time  SampleTime=-1
  V_FB : Constant  Value=k.V_FreeBoard
  cp_fg : Constant  Value=k.cp_fg
  cp_steel : Constant  Value=k.cp_steel
  p_amb : Constant  Value=k.p_amb
  T_fg_out : Outport  VectorParamsAs1DForOutWhenUnconnected=off
  Fi_fg_to_boiler : Outport  Port=2  VectorParamsAs1DForOutWhenUnconnected=off
  F_flyash_tot : Outport  Port=3  VectorParamsAs1DForOutWhenUnconnected=off
  wires:
  T_in/1 -> DIFF_Free Board/4(T_in)  "T_in"
  p_amb/1 -> DIFF_Free Board/8(p_amb)
  DIFF_Free Board/1(dMfg_dt_int) -> M_fg_part/1
  DIFF_Free Board/2(dTfg_dt) -> T_fg/1
  M_fg_part/1 -> DIFF_Free Board/1(M_fg_int)
  DIFF_Free Board/4(M_fg) -> Scope/1
  Q_rad/1 -> DIFF_Free Board/7(Q_rad)  "Q_rad"
  Fi_in/1 -> DIFF_Free Board/3(Fi_in)
  DIFF_Free Board/5(Y_H2O) -> To Workspace/1
  T_fg/1 -> DIFF_Free Board/2(T_fg), T_fg_out/1
  DIFF_Free Board/3(Fi_fg_out) -> Fi_fg_to_boiler/1
  V_FB/1 -> DIFF_Free Board/9(V_FreeBoard)
  Mw_gas/1 -> DIFF_Free Board/10(Mw_gas)
  T_amb/1 -> DIFF_Free Board/11(T_amb)
  cp_fg/1 -> DIFF_Free Board/12(cp_fg)
  cp_steel/1 -> DIFF_Free Board/13(cp_steel)
  M_steel/1 -> DIFF_Free Board/14(M_steel_FB)
  F_flyash_cell/1 -> Sum of Elements/1
  Sum of Elements/1 -> F_flyash_tot/1
  F_aII_in/1 -> DIFF_Free Board/5(F_aII)
  T_aII_in/1 -> DIFF_Free Board/6(T_aII)

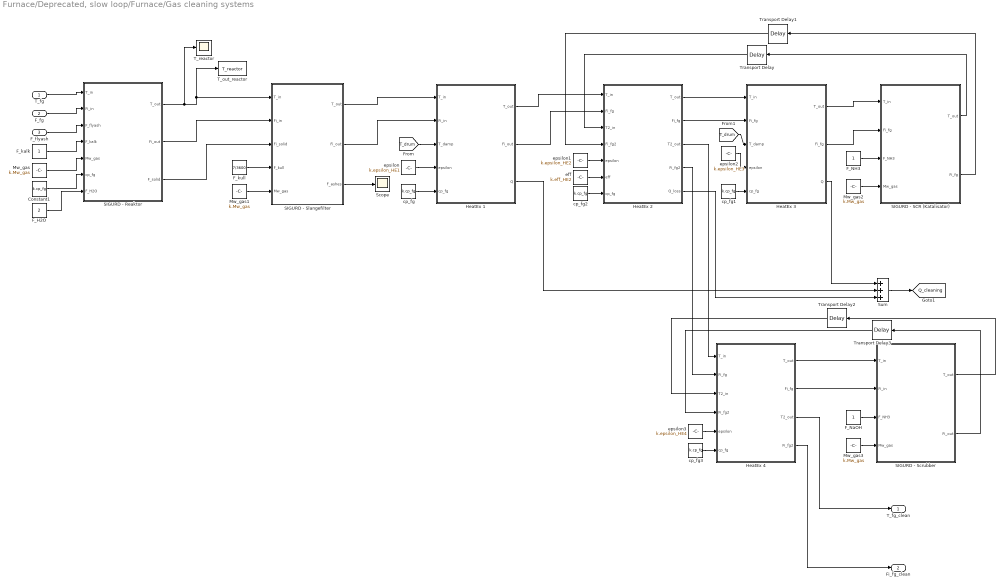
== system Furnace/Deprecated, slow loop/Furnace/Gas cleaning systems ==
  T_fg : Inport
  F_fg : Inport  Port=2
  F_flyash : Inport  Port=3
  Constant1 : Constant  Value=k.cp_fg
  F_H2O : Constant  Value=2
  F_NH3 : Constant
  F_NaOH : Constant
  F_kalk : Constant
  F_kull : Constant  Value=7/3600
  HeatEx 1 : MATLAB Function  TreatAsAtomicUnit=on
  HeatEx 2 : MATLAB Function  TreatAsAtomicUnit=on
  HeatEx 3 : MATLAB Function  TreatAsAtomicUnit=on
  HeatEx 4 : MATLAB Function  TreatAsAtomicUnit=on
  Mw_gas{,1..3} (4 alike) : Constant  Value=k.Mw_gas
  SIGURD - Reaktor : MATLAB Function  TreatAsAtomicUnit=on
  SIGURD - SCR (Katalisator) : MATLAB Function  TreatAsAtomicUnit=on
  SIGURD - Scrubber : MATLAB Function  TreatAsAtomicUnit=on
  SIGURD - Slangefilter : MATLAB Function  TreatAsAtomicUnit=on
  Scope : Scope
  Sum : Sum  Inputs=+++
  T_out_reactor : ToWorkspace  VariableName=T_reactor  SaveFormat=Timeseries  SampleTime=-1
  T_reactor : Scope
  Transport Delay : TransportDelay  DelayTime=2  InitialOutput=k.T_amb
  Transport Delay1 : TransportDelay  DelayTime=2  InitialOutput=ones(k.nc_gas,1)
  Transport Delay2 : TransportDelay  DelayTime=2  InitialOutput=k.T_amb
  Transport Delay3 : TransportDelay  DelayTime=2  InitialOutput=ones(k.nc_gas,1)
  cp_fg{,1..3} (4 alike) : Constant  Value=k.cp_fg
  eff : Constant  Value=k.eff_HE2
  epsilon : Constant  Value=k.epsilon_HE1
  epsilon1 : Constant  Value=k.epsilon_HE2
  epsilon2 : Constant  Value=k.epsilon_HE3
  epsilon3 : Constant  Value=k.epsilon_HE4
  T_fg_clean : Outport  VectorParamsAs1DForOutWhenUnconnected=off
  Fi_fg_clean : Outport  Port=2  VectorParamsAs1DForOutWhenUnconnected=off
  tag scope: Q_cleaning=global
  wires:
  T_fg/1 -> SIGURD - Reaktor/1(T_in)
  F_fg/1 -> SIGURD - Reaktor/2(Fi_in)
  SIGURD - Reaktor/1(T_out) -> T_reactor/1, T_out_reactor/1, SIGURD - Slangefilter/1(T_in)
  SIGURD - Reaktor/2(Fi_out) -> SIGURD - Slangefilter/2(Fi_in)
  F_kalk/1 -> SIGURD - Reaktor/4(F_kalk)
  Mw_gas/1 -> SIGURD - Reaktor/5(Mw_gas)
  F_kull/1 -> SIGURD - Slangefilter/4(F_kull)
  Mw_gas1/1 -> SIGURD - Slangefilter/5(Mw_gas)
  SIGURD - Slangefilter/1(T_out) -> HeatEx 1/1(T_in)
  SIGURD - Slangefilter/2(Fi_out) -> HeatEx 1/2(Fi_in)
  [T_drum] -> HeatEx 1/3(T_damp)
  epsilon/1 -> HeatEx 1/4(epsilon)
  HeatEx 1/1(T_out) -> HeatEx 2/1(T_in)
  HeatEx 1/2(Fi_out) -> HeatEx 2/2("Fi_fg ")
  HeatEx 2/1(T_out) -> HeatEx 3/1(T_in)
  HeatEx 2/2(Fi_fg) -> HeatEx 3/2("Fi_fg ")
  [T_drum] -> HeatEx 3/3(T_damp)
  epsilon1/1 -> HeatEx 2/5(epsilon)
  epsilon2/1 -> HeatEx 3/4(epsilon)
  HeatEx 1/3(Q) -> Sum/2
  HeatEx 3/3(Q) -> Sum/1
  HeatEx 3/1(T_out) -> SIGURD - SCR (Katalisator)/1(T_in)
  HeatEx 3/2(Fi_fg) -> SIGURD - SCR (Katalisator)/2("Fi_fg ")
  F_NH3/1 -> SIGURD - SCR (Katalisator)/3(F_NH3)
  Mw_gas2/1 -> SIGURD - SCR (Katalisator)/4(Mw_gas)
  SIGURD - SCR (Katalisator)/1(T_out) -> Transport Delay/1
  SIGURD - SCR (Katalisator)/2(Fi_fg) -> Transport Delay1/1
  HeatEx 2/3(T2_out) -> HeatEx 4/1(T_in)
  HeatEx 2/4(Fi_fg2) -> HeatEx 4/2("Fi_fg ")
  epsilon3/1 -> HeatEx 4/5(epsilon)
  HeatEx 4/1(T_out) -> SIGURD - Scrubber/1(T_in)
  HeatEx 4/2(Fi_fg) -> SIGURD - Scrubber/2(Fi_in)
  SIGURD - Scrubber/1(T_out) -> Transport Delay2/1
  SIGURD - Scrubber/2(Fi_out) -> Transport Delay3/1
  F_NaOH/1 -> SIGURD - Scrubber/3(F_NH3)
  Mw_gas3/1 -> SIGURD - Scrubber/4(Mw_gas)
  HeatEx 4/3(T2_out) -> T_fg_clean/1
  HeatEx 4/4(Fi_fg2) -> Fi_fg_clean/1
  SIGURD - Slangefilter/3(F_ashes) -> Scope/1
  cp_fg/1 -> HeatEx 1/5(cp_fg)
  cp_fg1/1 -> HeatEx 3/5(cp_fg)
  cp_fg2/1 -> HeatEx 2/7(cp_fg)
  Constant1/1 -> SIGURD - Reaktor/6(cp_fg)
  SIGURD - Reaktor/3(F_solid) -> SIGURD - Slangefilter/3(Fi_solid)
  F_flyash/1 -> SIGURD - Reaktor/3(F_flyash)
  Transport Delay/1 -> HeatEx 2/3(T2_in)
  Transport Delay1/1 -> HeatEx 2/4("Fi_fg2 ")
  Transport Delay2/1 -> HeatEx 4/3(T2_in)
  Transport Delay3/1 -> HeatEx 4/4("Fi_fg2 ")
  cp_fg3/1 -> HeatEx 4/6(cp_fg)
  eff/1 -> HeatEx 2/6(eff)
  Sum/1 -> [Q_cleaning]
  HeatEx 2/5(Q_loss) -> Sum/3
  F_H2O/1 -> SIGURD - Reaktor/7(F_H2O)

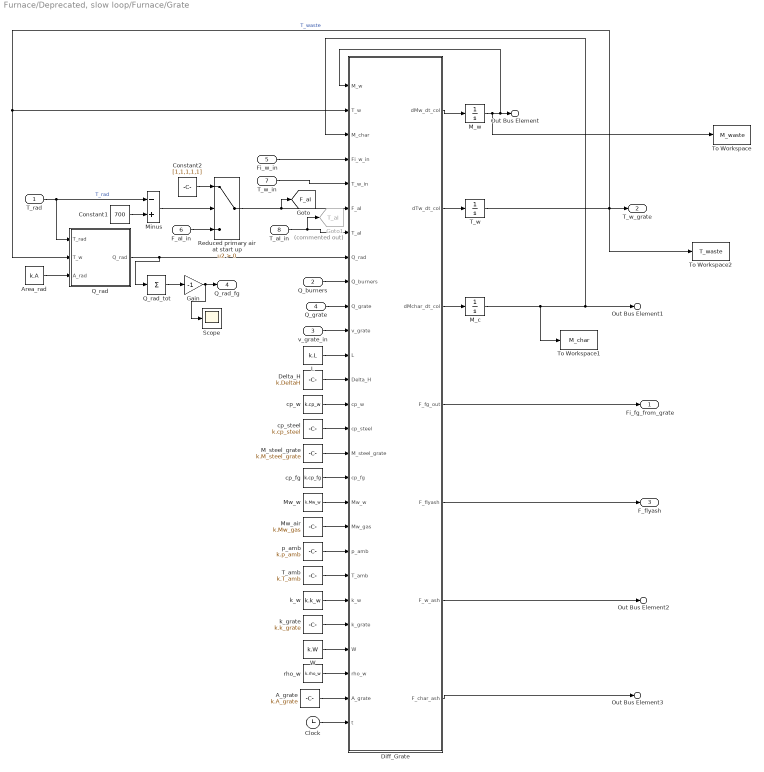
== system Furnace/Deprecated, slow loop/Furnace/Grate ==
  T_rad : Inport
  Q_burners : Inport  Port=2
  v_grate_in : Inport  Port=3
  Q_grate : Inport  Port=4
  Fi_w_in : Inport  Port=5
  F_aI_in : Inport  Port=6
  T_w_in : Inport  Port=7
  T_aI_in : Inport  Port=8
  A_grate : Constant  Value=k.A_grate
  Area_rad : Constant  Value=k.A
  Clock : Clock
  Constant1 : Constant  Value=700
  Constant2 : Constant  Value=[1,1,1,1,1]
  Delta_H : Constant  Value=k.DeltaH
  Diff_Grate : MATLAB Function  TreatAsAtomicUnit=on
  Gain : Gain  Gain=-1
  Goto1 : Goto  Commented=on  GotoTag=T_aI  TagVisibility=global
  L : Constant  Value=k.L
  M_c : Integrator  InitialCondition=zeros(k.n_cell,1)
  M_steel_grate : Constant  Value=k.M_steel_grate
  M_w : Integrator  InitialCondition=zeros(k.n_cell.*(k.nc_w+2),1)
  Minus : Sum  Inputs=-+
  Mw_air : Constant  Value=k.Mw_gas
  Mw_w : Constant  Value=k.Mw_w
  Q_rad : Subsystem
  Q_rad_tot : Sum  Inputs=+
  Reduced primary air at start up : Switch  Criteria=u2 > Threshold
  Scope : Scope
  T_amb : Constant  Value=k.T_amb
  T_w : Integrator  InitialCondition=k.T_amb.*ones(k.n_cell,1)
  To Workspace : ToWorkspace  VariableName=M_waste  SaveFormat=Structure With Time  SampleTime=-1
  To Workspace1 : ToWorkspace  VariableName=M_char  SaveFormat=Structure With Time  SampleTime=-1
  To Workspace2 : ToWorkspace  VariableName=T_waste  SaveFormat=Structure With Time  SampleTime=-1
  W : Constant  Value=k.W
  cp_fg : Constant  Value=k.cp_fg
  cp_steel : Constant  Value=k.cp_steel
  cp_w : Constant  Value=k.cp_w
  k_grate : Constant  Value=k.k_grate
  k_w : Constant  Value=k.k_w
  p_amb : Constant  Value=k.p_amb
  rho_w : Constant  Value=k.rho_w
  Fi_fg_from_grate : Outport  VectorParamsAs1DForOutWhenUnconnected=off
  T_w_grate : Outport  Port=2  VectorParamsAs1DForOutWhenUnconnected=off
  F_flyash : Outport  Port=3  VectorParamsAs1DForOutWhenUnconnected=off
  Q_rad_fg : Outport  Port=4  VectorParamsAs1DForOutWhenUnconnected=off
  Out Bus Element : Outport  Port=5  VectorParamsAs1DForOutWhenUnconnected=off  PortName=OutBus  Element=M_w_grate
  Out Bus Element1 : Outport  Port=5  VectorParamsAs1DForOutWhenUnconnected=off  PortName=OutBus  Element=M_char
  Out Bus Element2 : Outport  Port=5  VectorParamsAs1DForOutWhenUnconnected=off  PortName=OutBus  Element=F_w_ash
  Out Bus Element3 : Outport  Port=5  VectorParamsAs1DForOutWhenUnconnected=off  PortName=OutBus  Element=F_char_ash
  tag scope: F_aI=global
  wires:
  Diff_Grate/2(dTw_dt_col) -> T_w/1
  Area_rad/1 -> Q_rad/3(A_rad)
  M_w/1 -> To Workspace/1, Out Bus Element/1, Diff_Grate/1(M_w)
  T_aI_in/1 -> Goto1/1, Diff_Grate/7(T_aI)
  Q_rad/1(Q_rad) -> Q_rad_tot/1, Diff_Grate/8(Q_rad)
  Diff_Grate/1(dMw_dt_col) -> M_w/1
  T_w/1 -> Diff_Grate/2(T_w), Q_rad/2(T_w), T_w_grate/1, To Workspace2/1  "T_waste"
  Diff_Grate/6(F_w_ash) -> Out Bus Element2/1
  Diff_Grate/4(F_fg_out) -> Fi_fg_from_grate/1
  Diff_Grate/3(dMchar_dt_col) -> M_c/1
  M_c/1 -> To Workspace1/1, Out Bus Element1/1, Diff_Grate/3(M_char)
  Diff_Grate/7(F_char_ash) -> Out Bus Element3/1
  Q_rad_tot/1 -> Gain/1
  Gain/1 -> Scope/1, Q_rad_fg/1
  Q_burners/1 -> Diff_Grate/9(Q_burners)
  Clock/1 -> Diff_Grate/27(t)
  Q_grate/1 -> Diff_Grate/10(Q_grate)
  T_rad/1 -> Minus/1, Q_rad/1(T_rad)  "T_rad"
  Constant1/1 -> Minus/2
  Minus/1 -> Reduced primary air at start up/2
  F_aI_in/1 -> Reduced primary air at start up/3
  Reduced primary air at start up/1 -> [F_aI], Diff_Grate/6(F_aI)
  Constant2/1 -> Reduced primary air at start up/1
  L/1 -> Diff_Grate/12(L)
  Delta_H/1 -> Diff_Grate/13(Delta_H)
  cp_w/1 -> Diff_Grate/14(cp_w)
  cp_steel/1 -> Diff_Grate/15(cp_steel)
  M_steel_grate/1 -> Diff_Grate/16(M_steel_grate)
  cp_fg/1 -> Diff_Grate/17(cp_fg)
  Mw_w/1 -> Diff_Grate/18(Mw_w)
  Mw_air/1 -> Diff_Grate/19(Mw_gas)
  p_amb/1 -> Diff_Grate/20(p_amb)
  T_amb/1 -> Diff_Grate/21(T_amb)
  k_w/1 -> Diff_Grate/22(k_w)
  k_grate/1 -> Diff_Grate/23(k_grate)
  W/1 -> Diff_Grate/24(W)
  rho_w/1 -> Diff_Grate/25(rho_w)
  A_grate/1 -> Diff_Grate/26(A_grate)
  Diff_Grate/5(F_flyash) -> F_flyash/1
  v_grate_in/1 -> Diff_Grate/11(v_grate)
  Fi_w_in/1 -> Diff_Grate/4(Fi_w_in)
  T_w_in/1 -> Diff_Grate/5(T_w_in)

== system Furnace/Deprecated, slow loop/Furnace/Hot water to district heating ==
  In1 : Inport
  T_district : Scope
  wires:
  In1/1 -> T_district/1

== system Furnace/Deprecated, slow loop/Furnace/Turbine ==
  T_SH : Inport
  F_SH : Inport  Port=2
  p_drum : Inport  Port=3
  Scope : Scope
  Sum : Sum
  Transport Delay1 : TransportDelay  DelayTime=3
  Transport Delay2 : TransportDelay  DelayTime=3
  Turbine : MATLAB Function  TreatAsAtomicUnit=on
  W_net : Scope
  eta_TURB : Constant  Value=k.eta_TURB
  p_HP : Constant  Value=k.p_HP
  p_LP : Constant  Value=k.p_LP
  F_turb : Outport  VectorParamsAs1DForOutWhenUnconnected=off
  wires:
  T_SH/1 -> Turbine/1(T_SH)
  Turbine/1(W_el) -> Transport Delay1/1
  p_drum/1 -> Turbine/3(p_drum)
  F_SH/1 -> Transport Delay2/1, Turbine/2(F_SH)
  p_LP/1 -> Turbine/5(p_LP)
  Transport Delay1/1 -> Sum/1
  Transport Delay2/1 -> F_turb/1
  p_HP/1 -> Turbine/4(p_HP)
  Turbine/2(Q_turb) -> Scope/1
  eta_TURB/1 -> Turbine/6(eta_TURB)
  [W_fan] -> Sum/2
  Sum/1 -> W_net/1

== system Furnace/Plant2/Boiler/Drum ==
  F_ECO : Inport
  Q_EVA : Inport  Port=2
  F_vap : Inport  Port=3
  T_ECO : Inport  Port=4
  Q_cleaning : Inport  Port=5
  Constant : Constant  Value=k.p_amb
  Constant1 : Constant  Value=k.T_amb
  Constant10 : Constant  Value=k.cp_fg
  Constant11 : Constant  Value=k.Mw_air
  Constant2 : Constant  Value=k.Mw_water
  Constant3 : Constant  Value=k.V_gas
  Constant5 : Constant  Value=k.cp_water
  Constant6 : Constant  Value=k.V_EVA
  Constant7 : Constant  Value=k.rho_water
  Constant8 : Constant  Value=k.M_steel
  Constant9 : Constant  Value=k.cp_steel
  "DIFF_Boiler " : MATLAB Function  TreatAsAtomicUnit=on
  DIFF_Boiler_2 : MATLAB Function  TreatAsAtomicUnit=on
  DIFF_Boiler_vap : MATLAB Function  TreatAsAtomicUnit=on
  Integrator : Integrator  InitialCondition=k.A_0
  Integrator1 : Integrator  InitialCondition=k.M_H2O
  Scope : Scope
  cp_w : Constant  Value=k.cp_water
  T_drum : Outport  VectorParamsAs1DForOutWhenUnconnected=off
  x_vap : Outport  Port=2  VectorParamsAs1DForOutWhenUnconnected=off
  p_drum : Outport  Port=3  PortDimensions=1  VectorParamsAs1DForOutWhenUnconnected=off
  wires:
  F_vap/1 -> "DIFF_Boiler "/3(F_SH)
  Q_EVA/1 -> "DIFF_Boiler "/1(Q_EVA)
  F_ECO/1 -> "DIFF_Boiler "/2(F_ECO)
  "DIFF_Boiler "/1(dA_dt) -> Integrator/1
  Integrator/1 -> DIFF_Boiler_2/1(A)
  DIFF_Boiler_vap/1(x_vap) -> x_vap/1
  DIFF_Boiler_2/2(p) -> DIFF_Boiler_vap/2(p), p_drum/1
  Constant/1 -> DIFF_Boiler_2/2(p_amb)
  Constant1/1 -> DIFF_Boiler_2/3(T_amb)
  Constant2/1 -> DIFF_Boiler_2/4(Mw_water), DIFF_Boiler_vap/3(Mw_water)
  Constant3/1 -> DIFF_Boiler_2/5(V_gas)
  Integrator1/1 -> DIFF_Boiler_vap/4(M_H2O), DIFF_Boiler_2/6(M_H2O)
  Constant5/1 -> DIFF_Boiler_2/7(cp_water)
  Constant6/1 -> DIFF_Boiler_2/8(V_EVA), DIFF_Boiler_vap/5(V_EVA)
  Constant7/1 -> DIFF_Boiler_2/9(rho_water), DIFF_Boiler_vap/6(rho_water)
  Constant8/1 -> DIFF_Boiler_2/10(M_steel)
  Constant9/1 -> DIFF_Boiler_2/11(cp_steel)
  Constant10/1 -> DIFF_Boiler_2/12(cp_fg)
  Constant11/1 -> DIFF_Boiler_2/13(Mw_air)
  T_ECO/1 -> "DIFF_Boiler "/4(T_ECO)
  DIFF_Boiler_2/1(T_drum) -> "DIFF_Boiler "/5(T_drum), DIFF_Boiler_vap/1(T_drum), T_drum/1
  Q_cleaning/1 -> "DIFF_Boiler "/6(Q_cleaning)
  cp_w/1 -> "DIFF_Boiler "/7(cp_water)
  "DIFF_Boiler "/2(dM_dt) -> Integrator1/1, Scope/1
